simulink model "MotorControlSim_r2025b"  (R2025b)
settings: Solver=ode4  StartTime=0.0  StopTime=3  FixedStep=1e-5  RelTol=1e-3  EnableMultiTasking=on
values from neighbouring files (symbols this model uses):
  FOC_Ki = 121.716134791628    [MotorControlParameters.sldd]
  FOC_Kp = 0.0443190472886059    [MotorControlParameters.sldd]
  PMSM_B = 0.000861    [MotorControlParameters.sldd]
  PMSM_J = 0.000129    [MotorControlParameters.sldd]
  Vdc = 35.0    [MotorControlParameters.sldd]
libraries: MotorControlLibrary x12, slpidlib x2
settings Model: DataDictionary=MotorControlParameters.sldd  Creator=azmib  LastModifiedBy=tka008729
settings SolverCC: ZeroCrossControl=EnableAll  AutoInsertRateTranBlk=on  MaxZcPerStep=100.0
settings DataIOCC: SaveOutput=off  SaveTime=off
settings OptimizationCC: DefaultParameterBehavior=Inlined  InlineInvariantSignals=on  EnhancedBackFolding=on  PassReuseOutputArgsAs=Individual arguments  StateBitsets=on  DataBitsets=on  ZeroExternalMemoryAtStartup=off  ZeroInternalMemoryAtStartup=off  NoFixptDivByZeroProtection=on  LifeSpan=1  OptimizeBlockOrder=speed  DifferentSizesBufferReuse=on  EfficientTunableParamExpr=on
settings DebuggingCC: SignalInfNanChecking=error  ParameterTunabilityLossMsg=error
settings HardwareCC: ProdBitPerPointer=32.0  ProdBitPerSizeT=32.0  ProdBitPerPtrDiffT=32.0  ProdLargestAtomicFloat=None  ProdIntDivRoundTo=Floor  ProdWordSize=32.0  ProdHWDeviceType=Generic->Custom
settings SFSimCC: MATLABDynamicMemAlloc=off
settings RTWCC: SystemTargetFile=ert.tlc  TLCOptions=-p0  GenCodeOnly=on  TemplateMakefile=ert_default_tmf  GenerateReport=on  RTWVerbose=off  IncludeHyperlinkInReport=on  LaunchReport=on  Description=Embedded Coder
settings CodeAppCC: ForceParamTrailComments=on  IgnoreCustomStorageClasses=off  OperatorAnnotations=on  SimulinkDataObjDesc=on  SFDataObjDesc=on  CustomSymbolStrGlobalVar=rt$N$M  CustomSymbolStrType=$N$M  CustomSymbolStrFcn=$N$M$F  CustomSymbolStrMacro=$N$M  InsertBlockDesc=on
settings ERTTargetCC: RootIOFormat=Structure reference  ERTCustomFileTemplate=example_file_process.tlc  TargetLangStandard=C99 (ISO)  CodeReplacementLibrary=ISO_C  GenerateSampleERTMain=on  IncludeMdlTerminateFcn=off  SuppressErrorStatus=on  SupportAbsoluteTime=off  PurelyIntegerCode=on  SupportNonFinite=off  SupportComplex=off
settings SimscapeCC: SimscapeNominalValues="[{\"value\":\"1\",\"unit\":\"A\"},{\"value\":\"1\",\"unit\":\"bar\"},{\"value\":\"1\",\"unit\":\"cm^2\"},{\"value\":\"1\",\"unit\":\"cm^3/s\"},{\"value\":\"1\",\"unit\":\"kJ/kg\"},{\"value\":\"1\",\"unit\":\"kW\"},{\"value\":\"1\",\"unit\":\"l\"},{\"value\":\"1\",\"unit\":\"N\"},{\"value\":\"1\",\"unit\":\"N*m\"},{\"value\":\"1\",\"unit\":\"V\"},{\"value\":\"0.001\",\"unit\":\"Wb\"}]"  SimscapeLogType=all  SimscapeLogDataHistory=10000.0

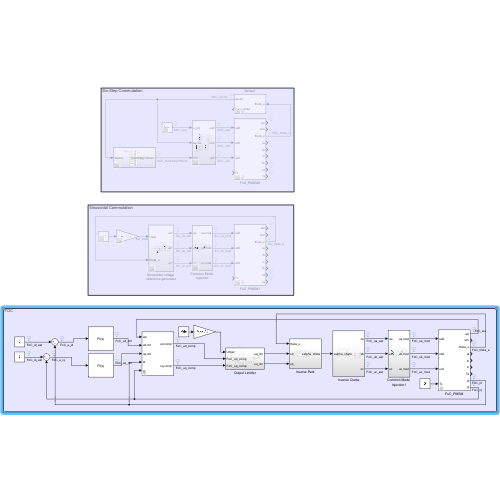
[thumbnail: Simulink's stored preview of the top-level diagram]
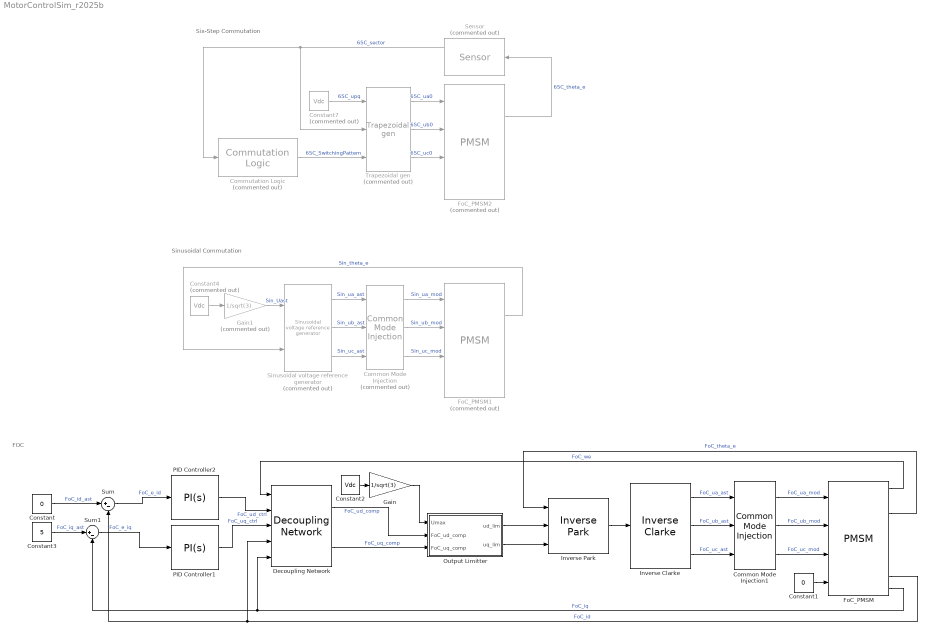
== system MotorControlSim_r2025b ==
  note: FOC
  note: Sinusoidal Commutation
  note: Six-Step Commutation
  Common Mode Injection : MotorControlLibrary/Common Mode  Injection  Commented=on  SystemSampleTime=-1  VariantActivationTime=update diagram  EmptyChoice=off  PassThrough=off  PassThroughVariantControl=(default)  EmptyChoiceVariantControl=(default)  AllowFlexibleInterface=on  Latency=0  AutoFrameSizeCalculation=off
  Common Mode Injection1 : MotorControlLibrary/Common Mode  Injection  SystemSampleTime=-1  VariantActivationTime=update diagram  EmptyChoice=off  PassThrough=off  PassThroughVariantControl=(default)  EmptyChoiceVariantControl=(default)  AllowFlexibleInterface=on  Latency=0  AutoFrameSizeCalculation=off
  Commutation Logic : MotorControlLibrary/Commutation Logic  Commented=on  SystemSampleTime=-1  VariantActivationTime=update diagram  EmptyChoice=off  PassThrough=off  PassThroughVariantControl=(default)  EmptyChoiceVariantControl=(default)  AllowFlexibleInterface=on  Latency=0  AutoFrameSizeCalculation=off
  Constant : Constant  Value=0
  Constant1 : Constant  Value=0
  Constant2 : Constant  Value=Vdc
  Constant3 : Constant  Value=5
  Constant4 : Constant  Commented=on  Value=Vdc
  Constant7 : Constant  Commented=on  Value=Vdc
  Decoupling Network : MotorControlLibrary/Decoupling Network  Ls=PMSM_Ls  psi_PM=PMSM_psiPM
  FoC_PMSM : MotorControlLibrary/PMSM  Rs=PMSM_Rs  Ls=PMSM_Ls  psi_PM=PMSM_psiPM  p=PMSM_p  J=PMSM_J  B=PMSM_B
  FoC_PMSM1 : MotorControlLibrary/PMSM  Commented=on  Rs=PMSM_Rs  Ls=PMSM_Ls  psi_PM=PMSM_psiPM  p=PMSM_p  J=PMSM_J  B=PMSM_B
  FoC_PMSM2 : MotorControlLibrary/PMSM  Commented=on  Rs=PMSM_Rs  Ls=PMSM_Ls  psi_PM=PMSM_psiPM  p=PMSM_p  J=PMSM_J  B=PMSM_B
  Gain : Gain  Gain=1/sqrt(3)
  Gain1 : Gain  Commented=on  Gain=1/sqrt(3)
  Inverse Clarke : MotorControlLibrary/Inverse Clarke  SystemSampleTime=-1  VariantActivationTime=update diagram  EmptyChoice=off  PassThrough=off  PassThroughVariantControl=(default)  EmptyChoiceVariantControl=(default)  AllowFlexibleInterface=on  Latency=0  AutoFrameSizeCalculation=off
  Inverse Park : MotorControlLibrary/Inverse Park  SystemSampleTime=-1  VariantActivationTime=update diagram  EmptyChoice=off  PassThrough=off  PassThroughVariantControl=(default)  EmptyChoiceVariantControl=(default)  AllowFlexibleInterface=on  Latency=0  AutoFrameSizeCalculation=off
  Output Limitter : Subsystem
  PID Controller1 : slpidlib/PID Controller  Controller=PI  Form=Parallel  TimeDomain=Continuous-time  UseExternalTs=off  SampleTime=-1  IntegratorMethod=Forward Euler  FilterMethod=Forward Euler  ControllerParametersSource=internal  P=FOC_Kp  I=FOC_Ki  UseKiTs=off  D=0  UseExternalDerivativeSource=off  N=100  UseFilter=on  TunerSelectOption=Transfer Function Based (PID Tuner App)  InitialConditionSource=internal  InitialConditionForIntegrator=0  InitialConditionForFilter=0  DifferentiatorICPrevScaledInput=0  ExternalReset=none  TrackingMode=off  Kt=1  LimitOutput=off  SatLimitsSource=external  UpperSaturationLimit=20.2  LowerSaturationLimit=-20.2  LinearizeAsGain=on  AntiWindupMode=back-calculation  Kb=1  LimitIntegrator=off  UpperIntegratorSaturationLimit=inf  LowerIntegratorSaturationLimit=-inf  POutMin=[]  POutMax=[]  IOutMin=[]  IOutMax=[]  DOutMin=[]  DOutMax=[]  NOutMin=[]  NOutMax=[]  SumOutMin=[]  SumOutMax=[]  SaturationOutMin=[]  SaturationOutMax=[]  PParamMin=[]  PParamMax=[]  IParamMin=[]  IParamMax=[]  DParamMin=[]  DParamMax=[]  NParamMin=[]  NParamMax=[]  KbParamMin=[]  KbParamMax=[]  KtParamMin=[]  KtParamMax=[]  KbOutMin=[]  KbOutMax=[]  KtOutMin=[]  KtOutMax=[]  IntegratorOutMin=[]  IntegratorOutMax=[]  FilterOutMin=[]  FilterOutMax=[]  SumI1OutMin=[]  SumI1OutMax=[]  SumI2OutMin=[]  SumI2OutMax=[]  SumI3OutMin=[]  SumI3OutMax=[]  SumI4OutMin=[]  SumI4OutMax=[]  SumDOutMin=[]  SumDOutMax=[]  DifferentiatorOutMin=[]  DifferentiatorOutMax=[]  FilterDiffOutCoefMin=[]  FilterDiffOutCoefMax=[]  ReciprocalOutMin=[]  ReciprocalOutMax=[]  SumDenOutMin=[]  SumDenOutMax=[]  SumNumOutMin=[]  SumNumOutMax=[]  DivideOutMin=[]  DivideOutMax=[]  UdiffTsProdOutMin=[]  UdiffTsProdOutMax=[]  NTsProdOutMin=[]  NTsProdOutMax=[]  UintegralTsProdOutMin=[]  UintegralTsProdOutMax=[]  UngainTsProdOutMin=[]  UngainTsProdOutMax=[]  ClampingZeroOutDataTypeStr=Inherit: Inherit via back propagation  ClampingZeroOutMin=[]  ClampingZeroOutMax=[]  FilterDenConstantOutDataTypeStr=Inherit: Inherit via back propagation  FilterDenConstantOutMin=[]  FilterDenConstantOutMax=[]  PCopyOutDataTypeStr=Inherit: Inherit via back propagation  PCopyOutMin=[]  PCopyOutMax=[]  NCopyOutDataTypeStr=Inherit: Inherit via back propagation  NCopyOutMin=[]  NCopyOutMax=[]  IntegratorContinuousStateAttributes=''  IntegratorStateMustResolveToSignalObject=off  IntegratorRTWStateStorageClass=Auto  FilterContinuousStateAttributes=''  FilterStateMustResolveToSignalObject=off  FilterRTWStateStorageClass=Auto  ParallelPVariant=InternalParameters  IdealPVariant=Disabled  IVariant=InternalParameters  DVariant=Disabled  IntegratorVariant=Continuous  SatVariant=Disabled  AWVariant=Passthrough  PCopyVariant=Disabled  TRVariant=Disabled  FdbkBlocksVariant=Forward  IdealPFdbkVariant=Disabled  SatFdbkVariant=Disabled  DerivativeFilterVariant=Disabled  NVariant=Disabled  NCopyVariant=Disabled_SignalSpec  FilterICVariant=Disabled  IntegratorICVariant=InternalICs  ExternalResetVariant=Disabled  TRSumVariant=Passthrough  SumFdbkVariant=Disabled  SumVariant=Sum_PI  TsampFilterVariant=InternalTs  TsampNgainVariant=Passthrough  TsampIntegralVariant=Disabled_SignalSpec  ExternalSaturationOutDataTypeStr=Inherit: Same as second input  DerivativeSourceVariant=Disabled  PreIntVariant=InternalPreInt
  PID Controller2 : slpidlib/PID Controller  Controller=PI  Form=Parallel  TimeDomain=Continuous-time  UseExternalTs=off  SampleTime=-1  IntegratorMethod=Forward Euler  FilterMethod=Forward Euler  ControllerParametersSource=internal  P=FOC_Kp  I=FOC_Ki  UseKiTs=off  D=0  UseExternalDerivativeSource=off  N=100  UseFilter=on  TunerSelectOption=Transfer Function Based (PID Tuner App)  InitialConditionSource=internal  InitialConditionForIntegrator=0  InitialConditionForFilter=0  DifferentiatorICPrevScaledInput=0  ExternalReset=none  TrackingMode=off  Kt=1  LimitOutput=off  SatLimitsSource=external  UpperSaturationLimit=20.2  LowerSaturationLimit=-20.2  LinearizeAsGain=on  AntiWindupMode=back-calculation  Kb=1  LimitIntegrator=off  UpperIntegratorSaturationLimit=inf  LowerIntegratorSaturationLimit=-inf  POutMin=[]  POutMax=[]  IOutMin=[]  IOutMax=[]  DOutMin=[]  DOutMax=[]  NOutMin=[]  NOutMax=[]  SumOutMin=[]  SumOutMax=[]  SaturationOutMin=[]  SaturationOutMax=[]  PParamMin=[]  PParamMax=[]  IParamMin=[]  IParamMax=[]  DParamMin=[]  DParamMax=[]  NParamMin=[]  NParamMax=[]  KbParamMin=[]  KbParamMax=[]  KtParamMin=[]  KtParamMax=[]  KbOutMin=[]  KbOutMax=[]  KtOutMin=[]  KtOutMax=[]  IntegratorOutMin=[]  IntegratorOutMax=[]  FilterOutMin=[]  FilterOutMax=[]  SumI1OutMin=[]  SumI1OutMax=[]  SumI2OutMin=[]  SumI2OutMax=[]  SumI3OutMin=[]  SumI3OutMax=[]  SumI4OutMin=[]  SumI4OutMax=[]  SumDOutMin=[]  SumDOutMax=[]  DifferentiatorOutMin=[]  DifferentiatorOutMax=[]  FilterDiffOutCoefMin=[]  FilterDiffOutCoefMax=[]  ReciprocalOutMin=[]  ReciprocalOutMax=[]  SumDenOutMin=[]  SumDenOutMax=[]  SumNumOutMin=[]  SumNumOutMax=[]  DivideOutMin=[]  DivideOutMax=[]  UdiffTsProdOutMin=[]  UdiffTsProdOutMax=[]  NTsProdOutMin=[]  NTsProdOutMax=[]  UintegralTsProdOutMin=[]  UintegralTsProdOutMax=[]  UngainTsProdOutMin=[]  UngainTsProdOutMax=[]  ClampingZeroOutDataTypeStr=Inherit: Inherit via back propagation  ClampingZeroOutMin=[]  ClampingZeroOutMax=[]  FilterDenConstantOutDataTypeStr=Inherit: Inherit via back propagation  FilterDenConstantOutMin=[]  FilterDenConstantOutMax=[]  PCopyOutDataTypeStr=Inherit: Inherit via back propagation  PCopyOutMin=[]  PCopyOutMax=[]  NCopyOutDataTypeStr=Inherit: Inherit via back propagation  NCopyOutMin=[]  NCopyOutMax=[]  IntegratorContinuousStateAttributes=''  IntegratorStateMustResolveToSignalObject=off  IntegratorRTWStateStorageClass=Auto  FilterContinuousStateAttributes=''  FilterStateMustResolveToSignalObject=off  FilterRTWStateStorageClass=Auto  ParallelPVariant=InternalParameters  IdealPVariant=Disabled  IVariant=InternalParameters  DVariant=Disabled  IntegratorVariant=Continuous  SatVariant=Disabled  AWVariant=Passthrough  PCopyVariant=Disabled  TRVariant=Disabled  FdbkBlocksVariant=Forward  IdealPFdbkVariant=Disabled  SatFdbkVariant=Disabled  DerivativeFilterVariant=Disabled  NVariant=Disabled  NCopyVariant=Disabled_SignalSpec  FilterICVariant=Disabled  IntegratorICVariant=InternalICs  ExternalResetVariant=Disabled  TRSumVariant=Passthrough  SumFdbkVariant=Disabled  SumVariant=Sum_PI  TsampFilterVariant=InternalTs  TsampNgainVariant=Passthrough  TsampIntegralVariant=Disabled_SignalSpec  ExternalSaturationOutDataTypeStr=Inherit: Same as second input  DerivativeSourceVariant=Disabled  PreIntVariant=InternalPreInt
  Sensor : MotorControlLibrary/Sensor  Commented=on  phi_e=SSC_phi_e
  Sinusoidal voltage reference generator : MotorControlLibrary/Sinusoidal voltage  reference generator  Commented=on  SystemSampleTime=-1  VariantActivationTime=update diagram  EmptyChoice=off  PassThrough=off  PassThroughVariantControl=(default)  EmptyChoiceVariantControl=(default)  AllowFlexibleInterface=on  Latency=0  AutoFrameSizeCalculation=off
  Sum : Sum  Inputs=|+-
  Sum1 : Sum  Inputs=|+-
  Trapezoidal gen : MotorControlLibrary/Trapezoidal gen  Commented=on  SystemSampleTime=-1  VariantActivationTime=update diagram  EmptyChoice=off  PassThrough=off  PassThroughVariantControl=(default)  EmptyChoiceVariantControl=(default)  AllowFlexibleInterface=on  Latency=0  AutoFrameSizeCalculation=off
  wires:
  Sensor/1 -> Commutation Logic/1, Trapezoidal gen/2  "6SC_sector"
  Commutation Logic/1 -> Trapezoidal gen/3  "6SC_SwitchingPattern"
  Trapezoidal gen/2 -> FoC_PMSM2/2  "6SC_ub0"
  Trapezoidal gen/1 -> FoC_PMSM2/1  "6SC_ua0"
  Trapezoidal gen/3 -> FoC_PMSM2/3  "6SC_uc0"
  FoC_PMSM2/3 -> Sensor/1  "6SC_theta_e"
  FoC_PMSM1/3 -> Sinusoidal voltage reference generator/2  "Sin_theta_e"
  Sinusoidal voltage reference generator/1 -> Common Mode Injection/1  "Sin_ua_ast"
  Sinusoidal voltage reference generator/2 -> Common Mode Injection/2  "Sin_ub_ast"
  Sinusoidal voltage reference generator/3 -> Common Mode Injection/3  "Sin_uc_ast"
  Common Mode Injection/1 -> FoC_PMSM1/1  "Sin_ua_mod"
  Common Mode Injection/2 -> FoC_PMSM1/2  "Sin_ub_mod"
  Common Mode Injection/3 -> FoC_PMSM1/3  "Sin_uc_mod"
  Inverse Clarke/2 -> Common Mode Injection1/2  "FoC_ub_ast"
  Inverse Clarke/1 -> Common Mode Injection1/1  "FoC_ua_ast"
  FoC_PMSM/3 -> Inverse Park/1  "FoC_theta_e"
  Inverse Clarke/3 -> Common Mode Injection1/3  "FoC_uc_ast"
  Inverse Park/1 -> Inverse Clarke/1
  Constant/1 -> Sum/1  "FoC_id_ast"
  Constant3/1 -> Sum1/1  "FoC_iq_ast"
  FoC_PMSM/1 -> Decoupling Network/1  "FoC_we"
  Gain1/1 -> Sinusoidal voltage reference generator/1  "Sin_Uast"
  Constant7/1 -> Trapezoidal gen/1  "6SC_upq"
  Common Mode Injection1/1 -> FoC_PMSM/1  "FoC_ua_mod"
  Common Mode Injection1/2 -> FoC_PMSM/2  "FoC_ub_mod"
  Common Mode Injection1/3 -> FoC_PMSM/3  "FoC_uc_mod"
  Sum/1 -> PID Controller2/1  "FoC_e_id"
  Sum1/1 -> PID Controller1/1  "FoC_e_iq"
  PID Controller2/1 -> Decoupling Network/2  "FoC_ud_ctrl"
  PID Controller1/1 -> Decoupling Network/3  "FoC_uq_ctrl"
  FoC_PMSM/8 -> Sum/2, Decoupling Network/4  "FoC_id"
  FoC_PMSM/9 -> Sum1/2, Decoupling Network/5  "FoC_iq"
  Constant1/1 -> FoC_PMSM/4
  Constant2/1 -> Gain/1
  Gain/1 -> Output Limitter/1(Umax)
  Decoupling Network/1 -> Output Limitter/2(FoC_ud_comp)  "FoC_ud_comp"
  Decoupling Network/2 -> Output Limitter/3(FoC_uq_comp)  "FoC_uq_comp"
  Output Limitter/1(ud_lim) -> Inverse Park/2
  Output Limitter/2(uq_lim) -> Inverse Park/3
  Constant4/1 -> Gain1/1

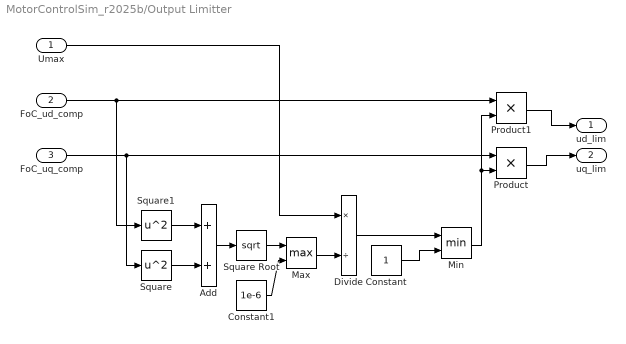
== system MotorControlSim_r2025b/Output Limitter ==
  Umax : Inport
  FoC_ud_comp : Inport  Port=2
  FoC_uq_comp : Inport  Port=3
  Add : Sum
  Constant : Constant
  Constant1 : Constant  Value=1e-6
  Divide : Product  Inputs=*/
  Max : MinMax  Function=max  Inputs=2
  Min : MinMax  Inputs=2
  Product : Product
  Product1 : Product
  Square : Math  Operator=square
  Square Root : Sqrt
  Square1 : Math  Operator=square
  ud_lim : Outport
  uq_lim : Outport  Port=2
  wires:
  FoC_ud_comp/1 -> Square1/1, Product1/1
  Min/1 -> Product1/2, Product/2
  Square/1 -> Add/2
  Square1/1 -> Add/1
  FoC_uq_comp/1 -> Square/1, Product/1
  Divide/1 -> Min/1
  Umax/1 -> Divide/1
  Product1/1 -> ud_lim/1
  Add/1 -> Square Root/1
  Product/1 -> uq_lim/1
  Constant/1 -> Min/2
  Max/1 -> Divide/2
  Square Root/1 -> Max/1
  Constant1/1 -> Max/2
